simulink model "lista1_6b"  (R2020b)
settings: Solver=VariableStepAuto  StartTime=0.0  StopTime=20  RelTol=1e-3
settings Model: Creator=lucas  LastModifiedBy=lucas

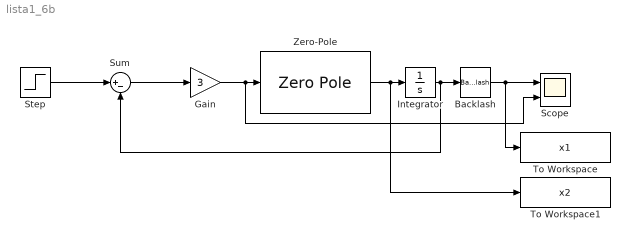
== system lista1_6b ==
  Backlash : Backlash
  Gain : Gain  Gain=3
  Integrator : Integrator
  Scope : Scope  NumInputPorts=2
  Step : Step  Time=0  SampleTime=0
  Sum : Sum  Inputs=|+-
  To Workspace : ToWorkspace  VariableName=x1  SaveFormat=Timeseries  SampleTime=-1
  To Workspace1 : ToWorkspace  VariableName=x2  SaveFormat=Timeseries  SampleTime=-1
  Zero-Pole : ZeroPole  Zeros=[]  Poles=[-1 -5]  Gain=5
  wires:
  Step/1 -> Sum/1
  Gain/1 -> Scope/2, Zero-Pole/1
  Integrator/1 -> Sum/2, Backlash/1
  Zero-Pole/1 -> To Workspace1/1, Integrator/1
  Sum/1 -> Gain/1
  Backlash/1 -> Scope/1, To Workspace/1
